simulink model "MIL_pos_pade_observer_discrete_antiwindup"  (R2023b)
settings: Solver=VariableStepAuto  StartTime=0.0  StopTime=40  FixedStep=Ts  RelTol=1e-3
values from neighbouring files (symbols this model uses):
  kr = -1/(C*inv(A-B*K_tilde(1:3))*B)    [controller_tuning.m]
  sys_discrete = c2d(sys_continuos,0.005,'tustin')    [observer.m]
undefined symbols (not defined in the file or in its folder): A, B, C, disturbance, K_tilde, Ts
libraries: cstblocks x2, eeStairGenerator x1
settings Model: Creator=giova  LastModifiedBy=giova

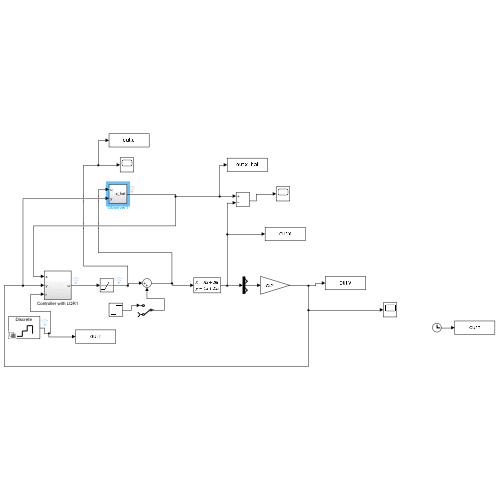
[thumbnail: Simulink's stored preview of the top-level diagram]
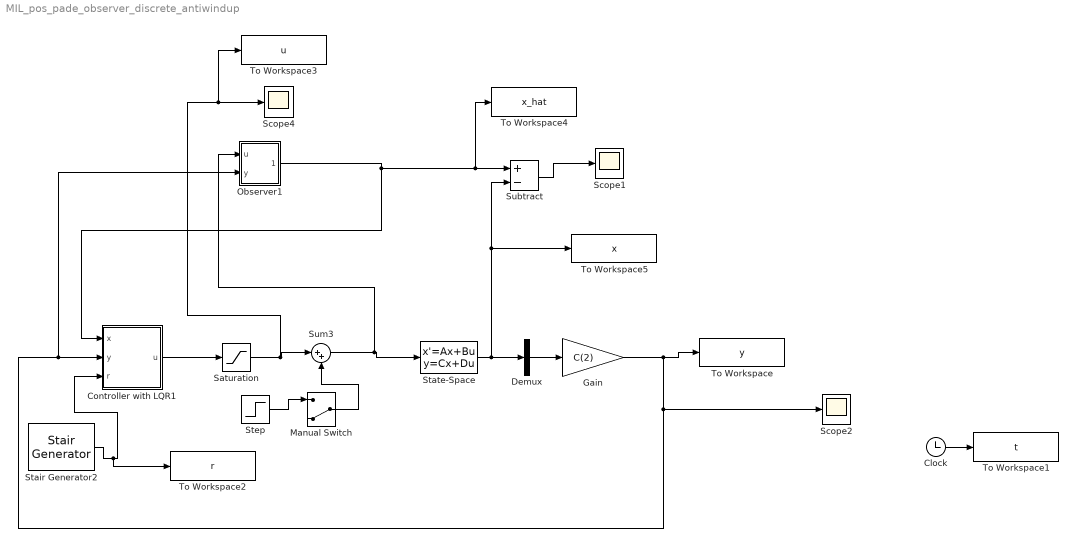
== system MIL_pos_pade_observer_discrete_antiwindup ==
  Clock : Clock
  Controller with LQR1 : Subsystem
  Demux : Demux  Outputs=3
  Gain : Gain  Gain=C(2)
  Manual Switch : ManualSwitch  CurrentSetting=0
  Observer1 : Subsystem
  Saturation : Saturate  UpperLimit=12  LowerLimit=-12
  Scope1 : Scope
  Scope2 : Scope
  Scope4 : Scope
  Stair Generator2 : eeStairGenerator/Stair Generator  LabelModeActiveChoice=Discrete  TimeInput=[0 10 20 30]  AmplitudeInput=[0 pi 2*pi pi/2]  SampleTime=Ts  RepeatPattern=off  OutDataTypeStr=double
      settings: LibrarySourceBlock=ee_sl_lib/General Control/Stair Generator
  State-Space : StateSpace  A=A  B=B  C=eye(3)  D=[0;0;0]  InitialCondition=0
  Step : Step  Time=2  After=disturbance  SampleTime=0
  Subtract : Sum  Inputs=+-
  Sum3 : Sum  Inputs=|++
  To Workspace : ToWorkspace  VariableName=y  SampleTime=Ts
      settings: Save2DSignal=2-D array (concatenate along first dimension)
  To Workspace1 : ToWorkspace  VariableName=t  SampleTime=Ts
      settings: Save2DSignal=2-D array (concatenate along first dimension)
  To Workspace2 : ToWorkspace  VariableName=r  SampleTime=Ts
      settings: Save2DSignal=2-D array (concatenate along first dimension)
  To Workspace3 : ToWorkspace  VariableName=u  SampleTime=Ts
      settings: Save2DSignal=2-D array (concatenate along first dimension)
  To Workspace4 : ToWorkspace  VariableName=x_hat  SampleTime=Ts
      settings: Save2DSignal=2-D array (concatenate along first dimension)
  To Workspace5 : ToWorkspace  VariableName=x  SampleTime=Ts
      settings: Save2DSignal=2-D array (concatenate along first dimension)
  wires:
  Controller with LQR1/1(u) -> Saturation/1
  Clock/1 -> To Workspace1/1
  Observer1/1(x_hat) -> Controller with LQR1/1(x), To Workspace4/1, Subtract/1
  Demux/2 -> Gain/1
  Subtract/1 -> Scope1/1
  Gain/1 -> Controller with LQR1/2(y), Observer1/2(y), Scope2/1, To Workspace/1
  State-Space/1 -> Demux/1, To Workspace5/1, Subtract/2
  Saturation/1 -> Scope4/1, To Workspace3/1, Sum3/1
  Stair Generator2/1 -> To Workspace2/1, Controller with LQR1/3(r)
  Step/1 -> Manual Switch/1
  Manual Switch/1 -> Sum3/2
  Sum3/1 -> Observer1/1(u), State-Space/1

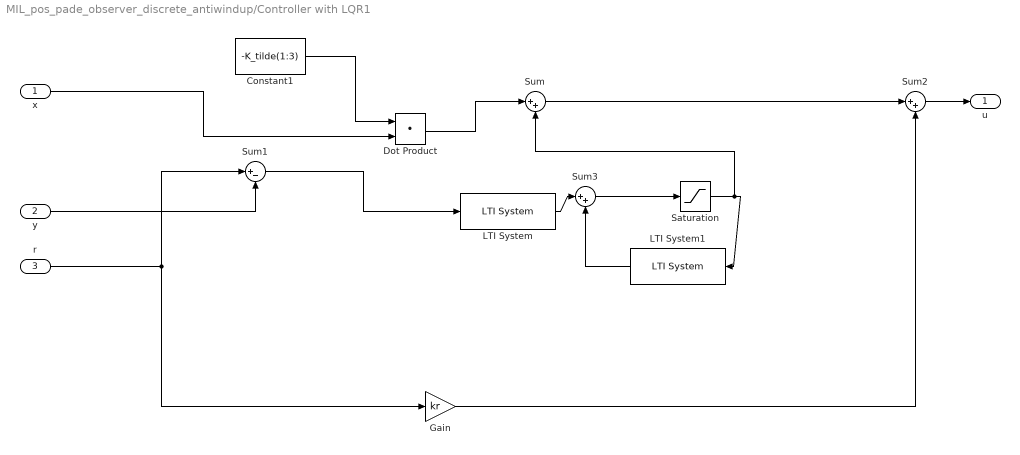
== system MIL_pos_pade_observer_discrete_antiwindup/Controller with LQR1 ==
  x : Inport
  y : Inport  Port=2
  r : Inport  Port=3
  Constant1 : Constant  Value=-K_tilde(1:3)
  Dot Product : DotProduct  OutDataTypeStr=Inherit: Inherit via internal rule
  Gain : Gain  Gain=kr
  LTI System : cstblocks/LTI System  sys=z_Q_Gamma  IC=[]  PadeOrder=0
  LTI System1 : cstblocks/LTI System  sys=z_antiwindupFunc  IC=[]  PadeOrder=0
  Saturation : Saturate  UpperLimit=12  LowerLimit=-12
  Sum : Sum  Inputs=|++
  Sum1 : Sum  Inputs=|+-
  Sum2 : Sum  Inputs=|++
  Sum3 : Sum  Inputs=|++
  u : Outport
  wires:
  Dot Product/1 -> Sum/1
  y/1 -> Sum1/2
  x/1 -> Dot Product/2
  Sum2/1 -> u/1
  Constant1/1 -> Dot Product/1
  r/1 -> Gain/1, Sum1/1
  Sum/1 -> Sum2/1
  Gain/1 -> Sum2/2
  LTI System/1 -> Sum3/1
  Sum3/1 -> Saturation/1
  Saturation/1 -> LTI System1/1, Sum/2
  LTI System1/1 -> Sum3/2
  Sum1/1 -> LTI System/1

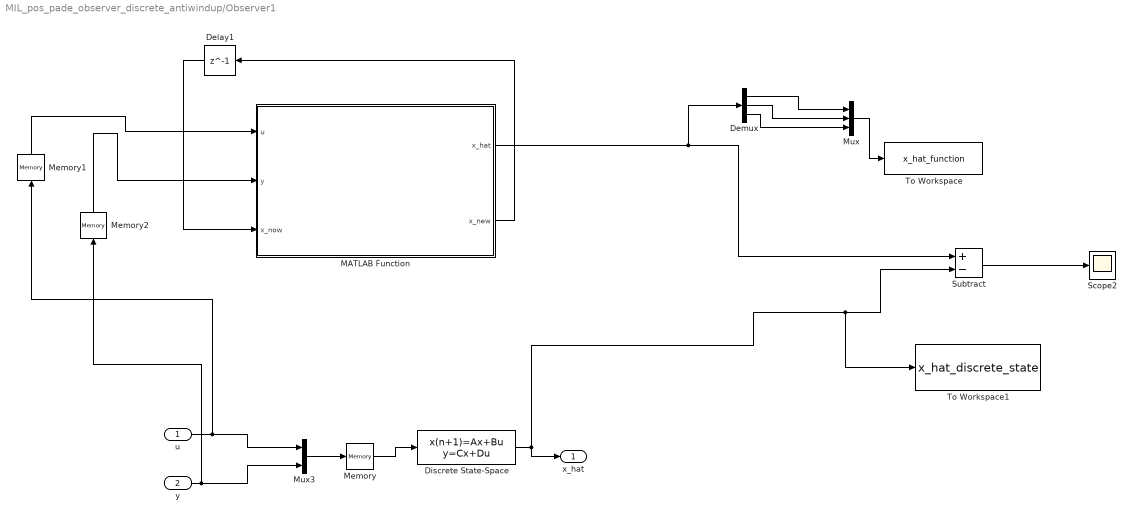
== system MIL_pos_pade_observer_discrete_antiwindup/Observer1 ==
  u : Inport
  y : Inport  Port=2
  Delay1 : Delay  DelayLength=1  InitialCondition=[0;0;0]  SampleTime=Ts
  Demux : Demux  Outputs=3
  Discrete State-Space : DiscreteStateSpace  A=sys_discrete.A  B=sys_discrete.B  C=sys_discrete.C  D=sys_discrete.D  SampleTime=Ts
  MATLAB Function : MATLAB Function  TreatAsAtomicUnit=on
  Memory : Memory  InitialCondition=[0;0]
  Memory1 : Memory
  Memory2 : Memory
  Mux : Mux  Inputs=3
  Mux3 : Mux  Inputs=2
  Scope2 : Scope
  Subtract : Sum  Inputs=+-
  To Workspace : ToWorkspace  VariableName=x_hat_function  SampleTime=Ts
      settings: Save2DSignal=2-D array (concatenate along first dimension)
  To Workspace1 : ToWorkspace  VariableName=x_hat_discrete_state  SampleTime=Ts
      settings: Save2DSignal=2-D array (concatenate along first dimension)
  x_hat : Outport
  wires:
  Memory1/1 -> MATLAB Function/1(u)
  Memory2/1 -> MATLAB Function/2(y)
  Subtract/1 -> Scope2/1
  MATLAB Function/1(x_hat) -> Demux/1, Subtract/1
  MATLAB Function/2(x_new) -> Delay1/1
  Memory/1 -> Discrete State-Space/1
  Discrete State-Space/1 -> To Workspace1/1, Subtract/2, x_hat/1
  Mux3/1 -> Memory/1
  u/1 -> Memory1/1, Mux3/1
  y/1 -> Memory2/1, Mux3/2
  Delay1/1 -> MATLAB Function/3(x_now)
  Demux/1 -> Mux/1
  Demux/2 -> Mux/2
  Demux/3 -> Mux/3
  Mux/1 -> To Workspace/1

== matlab function MIL_pos_pade_observer_discrete_antiwindup/Observer1/MATLAB Function ==
  data: u input; x_hat output; y input; x_new output; x_now input
function [x_hat,x_new]= fcn(u, y, x_now)
A = [0.931605363824459  -11.346656884140103    0.039099543321700;
    0.002741925544432    0.119498209981127    5.550203919352659e-05;
   -0.007094455468349   -2.896588572120294    0.837920445653216];

B = [-0.004047022543127    1.941673905307397;
   -5.744773077210588e-06    0.150674103104834;
    0.036776145051735    0.495672910737163];
    
C = [0.965802681912229  -5.673328442070051    0.019549771660850;
    0.001370962772216    0.559749104990563    2.775101959676330e-05;
   -0.003547227734175  -1.448294286060147    0.918960222826608];

D = [-0.002023511271564    0.970836952653698;
   -2.872386538605294e-06   0.075337051552417;
    0.018388072525868   0.247836455368581];

x1 = x_now(1);
x2 = x_now(2);
x3 = x_now(3);

x1_stimato = C(1) * x1 + C(4) * x2 + C(7) * x3 + D(1) * u + D(4) * y;
x2_stimato = C(2) * x1 + C(5) * x2 + C(8) * x3 + D(2) * u + D(5) * y;
x3_stimato = C(3) * x1 + C(6) * x2 + C(9) * x3 + D(3) * u + D(6) * y;

x1_new = A(1) * x1 + A(4) * x2 + A(7) * x3 + B(1) * u + B(4) * y;
x2_new = A(2) * x1 + A(5) * x2 + A(8) * x3 + B(2) * u + B(5) * y;
x3_new = A(3) * x1 + A(6) * x2 + A(9) * x3 + B(3) * u + B(6) * y;


x_new = [x1_new ;x2_new ;x3_new];
x_hat = [x1_stimato ;x2_stimato ;x3_stimato];
